simulink model "MLC_LQE_benchmarking_Model_2020b_students"  (R2020b)
settings: Solver=FixedStepAuto  StartTime=0.0  StopTime=Tend  FixedStep=dt  RelTol=1e-3
values from neighbouring files (symbols this model uses):
  cost_threshold = 1.5    [MLC_LQE_benchmarking_evaluator_students.m]    (also in MLC_LQR_benchmarking_evaluator_students.m = 1000)
  Init_cond_estMLC = C_estMLC_inv./(size(C_estMLC_inv,2)-size(idx_tmp,2))    [MLC_LQE_benchmarking_evaluator_students.m]
undefined symbols (not defined in the file or in its folder): A_estMLC, B_estMLC, C_estMLC, D_estMLC, dt, InitCond, sysOL, Vd, Vn
libraries: simulink x1
settings Model: Creator=mario  LastModifiedBy=mario

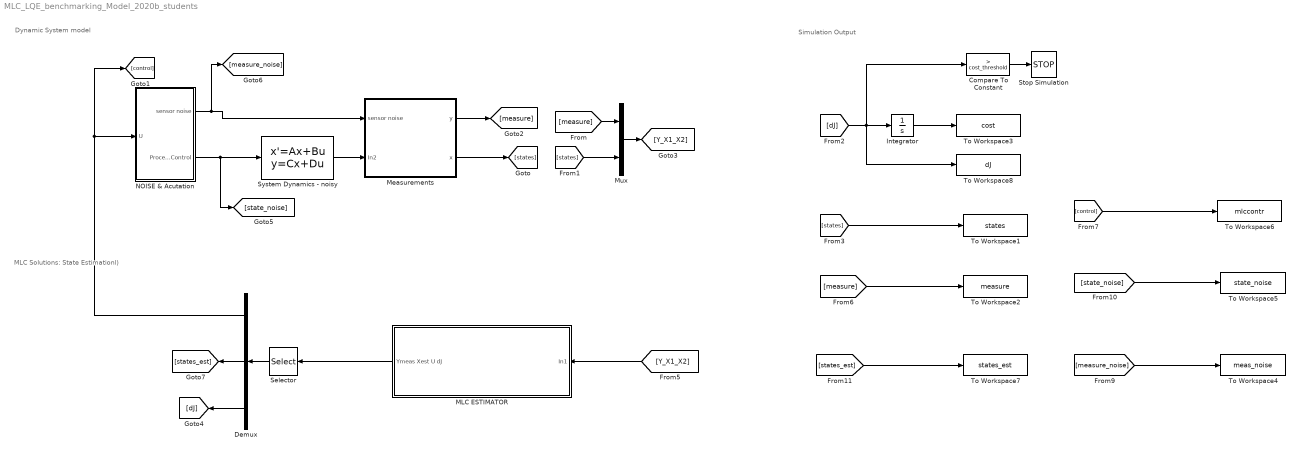
== system MLC_LQE_benchmarking_Model_2020b_students ==
  note: Dynamic System model
  note: MLC Solutions: State Estimationl)
  note: Simulation Output
  Compare To Constant : simulink/Logic and Bit Operations/Compare To Constant  relop=>  const=cost_threshold  OutDataTypeStr=boolean
  Demux : Demux  Outputs=[1 2 1]
  Integrator : Integrator
  MLC ESTIMATOR : Subsystem  TreatAsAtomicUnit=on
  Measurements : Subsystem
  Mux : Mux  Inputs=[1 2]
  NOISE & Acutation : Subsystem
  Selector : Selector  InputPortWidth=5  IndexOptions=Index vector (dialog)  Indices=[4 2 3 5]  OutputSizes=1
  Stop Simulation : Stop
  System Dynamics - noisy : StateSpace  A=sysOL.a  B=sysOL.b  C=eye(2)  D=[0 0 0; 0 0 0]  InitialCondition=InitCond
  To Workspace1 : ToWorkspace  VariableName=states  SaveFormat=Timeseries  SampleTime=-1
  To Workspace2 : ToWorkspace  VariableName=measure  SaveFormat=Timeseries  SampleTime=-1
  To Workspace3 : ToWorkspace  VariableName=cost  SaveFormat=Timeseries  SampleTime=-1
  To Workspace4 : ToWorkspace  VariableName=meas_noise  SaveFormat=Timeseries  SampleTime=-1
  To Workspace5 : ToWorkspace  VariableName=state_noise  SaveFormat=Timeseries  SampleTime=-1
  To Workspace6 : ToWorkspace  VariableName=mlccontr  SaveFormat=Timeseries  SampleTime=-1
  To Workspace7 : ToWorkspace  VariableName=states_est  SaveFormat=Timeseries  SampleTime=-1
  To Workspace8 : ToWorkspace  VariableName=dJ  SaveFormat=Timeseries  SampleTime=-1
  wires:
  NOISE & Acutation/2(ProcessNoiseControl) -> [state_noise], System Dynamics - noisy/1
  System Dynamics - noisy/1 -> Measurements/2(In2)
  Compare To Constant/1 -> Stop Simulation/1
  NOISE & Acutation/1(sensor noise) -> [measure_noise], Measurements/1(sensor noise)
  Demux/1 -> NOISE & Acutation/1(U), [control]
  Measurements/2(x) -> [states]
  Measurements/1(y) -> [measure]
  Integrator/1 -> To Workspace3/1
  [dJ] -> Compare To Constant/1, Integrator/1, To Workspace8/1
  [measure] -> Mux/1
  [states] -> Mux/2
  Mux/1 -> [Y_X1_X2]
  Selector/1 -> Demux/1
  [Y_X1_X2] -> MLC ESTIMATOR/1(In1)
  MLC ESTIMATOR/1(Ymeas Xest U dJ) -> Selector/1
  Demux/2 -> [states_est]
  [states] -> To Workspace1/1
  [measure] -> To Workspace2/1
  Demux/3 -> [dJ]
  [control] -> To Workspace6/1
  [measure_noise] -> To Workspace4/1
  [state_noise] -> To Workspace5/1
  [states_est] -> To Workspace7/1

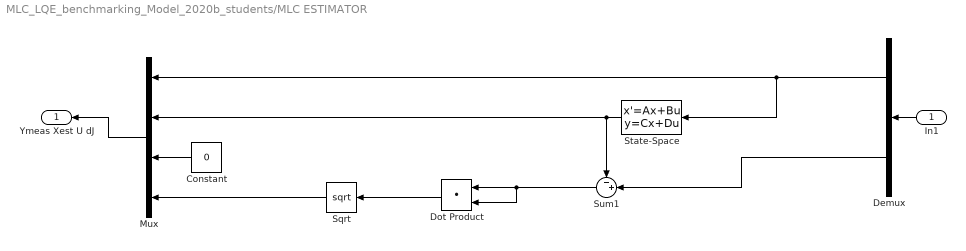
== system MLC_LQE_benchmarking_Model_2020b_students/MLC ESTIMATOR ==
  In1 : Inport
  Constant : Constant  Value=0
  Demux : Demux  Outputs=[1 2]
  Dot Product : DotProduct  InputSameDT=on  OutDataTypeStr=Inherit: Inherit via internal rule
  Mux : Mux  Inputs=[1 2 1 1]
  Sqrt : Sqrt  SaturateOnIntegerOverflow=on
  State-Space : StateSpace  A=A_estMLC  B=B_estMLC  C=C_estMLC  D=D_estMLC  InitialCondition=Init_cond_estMLC
  Sum1 : Sum  Inputs=-+|
  Ymeas Xest U dJ : Outport
  wires:
  Demux/2 -> Sum1/2
  In1/1 -> Demux/1
  Mux/1 -> Ymeas Xest U dJ/1
  Demux/1 -> Mux/1, State-Space/1
  State-Space/1 -> Sum1/1, Mux/2
  Constant/1 -> Mux/3
  Dot Product/1 -> Sqrt/1
  Sum1/1 -> Dot Product/2, Dot Product/1
  Sqrt/1 -> Mux/4

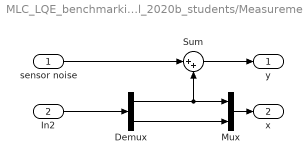
== system MLC_LQE_benchmarking_Model_2020b_students/Measurements ==
  sensor noise : Inport
  In2 : Inport  Port=2
  Demux : Demux  Outputs=2
  Mux : Mux  Inputs=2
  Sum : Sum  Inputs=|++
  y : Outport
  x : Outport  Port=2
  wires:
  Sum/1 -> y/1
  Demux/1 -> Sum/2, Mux/1
  Demux/2 -> Mux/2
  Mux/1 -> x/1
  sensor noise/1 -> Sum/1
  In2/1 -> Demux/1

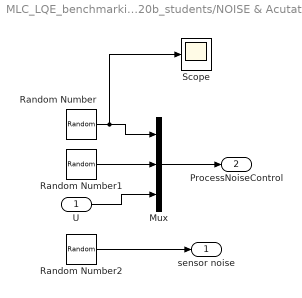
== system MLC_LQE_benchmarking_Model_2020b_students/NOISE & Acutation ==
  U : Inport
  Mux : Mux  Inputs=3
  Random Number : RandomNumber  Variance=Vd(1,1)^2  SampleTime=dt
  Random Number1 : RandomNumber  Variance=Vd(2,2)^2  SampleTime=dt
  Random Number2 : RandomNumber  Variance=Vn  SampleTime=dt
  Scope : Scope
  sensor noise : Outport
  ProcessNoiseControl : Outport  Port=2
  wires:
  Mux/1 -> ProcessNoiseControl/1
  Random Number2/1 -> sensor noise/1
  U/1 -> Mux/3
  Random Number/1 -> Mux/1, Scope/1
  Random Number1/1 -> Mux/2
